simulink library "lib_integrator"  (Simulink 7.7)
settings: Solver=ode45  StartTime=0.0  StopTime=10.0  RelTol=1e-3
undefined symbols (not defined in the file): T_veh, v0, v_max
settings Model: Creator=lfeng  LastModifiedBy=lfeng

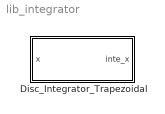
== system lib_integrator ==
  Disc_Integrator_Trapezoidal : Subsystem  mask{x0=v0, T=T_veh, upp_limit=v_max, low_limit=0}
      mask prompts: x0 "Initial value"; T "Sample time"; upp_limit "Upper saturation limit"; low_limit "Lower saturation limit"

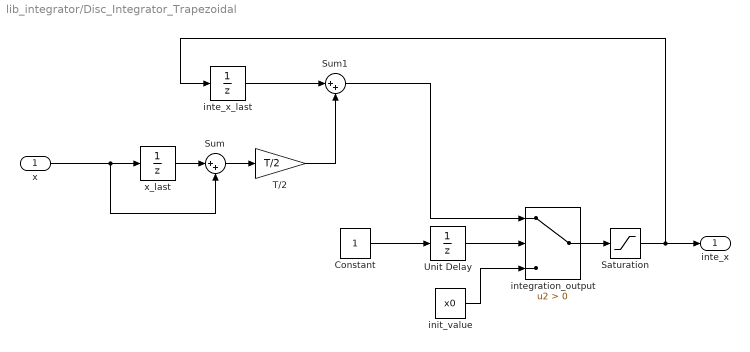
== system lib_integrator/Disc_Integrator_Trapezoidal ==
  x : Inport
  Constant : Constant  OutDataTypeStr=boolean
  Saturation : Saturate  UpperLimit=upp_limit  LowerLimit=low_limit
  Sum : Sum  Inputs=|++
  Sum1 : Sum  Inputs=|++
  T/2 : Gain  Gain=T/2
  Unit Delay : UnitDelay  SampleTime=-1
  init_value : Constant  Value=x0
  inte_x_last : UnitDelay  SampleTime=-1
  integration_output : Switch  Criteria=u2 > Threshold
  x_last : UnitDelay  SampleTime=-1
  inte_x : Outport
  wires:
  Saturation/1 -> inte_x/1, inte_x_last/1
  integration_output/1 -> Saturation/1
  init_value/1 -> integration_output/3
  Unit Delay/1 -> integration_output/2
  Constant/1 -> Unit Delay/1
  x/1 -> x_last/1, Sum/2
  x_last/1 -> Sum/1
  Sum/1 -> T/2/1
  inte_x_last/1 -> Sum1/1
  T/2/1 -> Sum1/2
  Sum1/1 -> integration_output/1
